simulink model "BatteryStoragePVPlantGFM"  (R2023a)
settings: Solver=FixedStepDiscrete  StartTime=0.0  StopTime=SimulationTime  RelTol=1e-3
PreLoadFcn:
  | run('BatteryStoragePVPlantGFMParameters')
undefined symbols (not defined in the file): Array, Base, battery, BatteryInverter, DiscIntNeverNeededParam, ee, Feeder, fRT, GFLBatteryController, GFMBatteryController, Grid, GridTransformer, Line, Load, Load2CB_final, Load2CB_initial, LVRT, maxSoC, maxVdc, minIrrad, minSoC, minVdc, Mpp, olTime, Panel, PVController, PVInverter, PVTransformer, Scenario, SM, SubTransmissionLine, Ts, VSMbase
libraries: ee_lib x51, nesl_utility x45, fl_lib x26, eeGeneralControl x18, simulink x12, eeTransforms x11, slpidlib x8, eePowerMeasurement x5, batteryecm_lib x2, eeTotalHarmonicDistorsion x2, spsLeadLagFilterLib x1, eeSmAC1C x1
(part 5 of 5)

== system BatteryStoragePVPlantGFM/BESS & PV PARK/60 MWhr Battery Energy Storage/Variant Subsystem/Grid Forming VSM/Battery Inverter B1/controller/GridFormingController/Current Limiting ==
  In Bus Element : Inport  PortName=measure  Element=Igd
  In Bus Element1 : Inport  PortName=measure  Element=Igq
  In Bus Element2 : Inport  Port=2  PortName=reactiveControl  Element=Vmd
  In Bus Element4 : Inport  Port=2  PortName=reactiveControl  Element=Vmq
  CurrentLimitingMethod : Subsystem  Variant=on  VariantControlMode=label  VariantControl=Choice  LabelModeActiveChoice=virimp
  Gain1 : Gain  Gain=1/(power/(sqrt(3)*girdLineVoltage)*sqrt(2/3))
  Gain5 : Gain  Gain=1/(power/(sqrt(3)*girdLineVoltage)*sqrt(2/3))
  Subtract : Sum  Inputs=+-
  Subtract1 : Sum  Inputs=-+
  Out Bus Element : Outport  PortName=currentLimiting  Element=Vmd
  Out Bus Element1 : Outport  PortName=currentLimiting  Element=Vmq
  Out Bus Element2 : Outport  PortName=currentLimiting  Element=Idmax
  Out Bus Element3 : Outport  PortName=currentLimiting  Element=Iqmax
  wires:
  In Bus Element/1 -> Gain5/1
  In Bus Element2/1 -> Subtract/1
  Gain1/1 -> CurrentLimitingMethod/2(Igq)
  In Bus Element4/1 -> Subtract1/2
  Subtract/1 -> Out Bus Element/1
  Subtract1/1 -> Out Bus Element1/1
  CurrentLimitingMethod/3(Idmax) -> Out Bus Element2/1
  CurrentLimitingMethod/4(Iqmax) -> Out Bus Element3/1
  Gain5/1 -> CurrentLimitingMethod/1(Igd)  "Q"
  In Bus Element1/1 -> Gain1/1
  CurrentLimitingMethod/1(delVmd) -> Subtract/2
  CurrentLimitingMethod/2(delVmq) -> Subtract1/1

== system BatteryStoragePVPlantGFM/BESS & PV PARK/60 MWhr Battery Energy Storage/Variant Subsystem/Grid Forming VSM/Battery Inverter B1/controller/GridFormingController/Measurement ==
  Vgabcc : Inport
  Igabc : Inport  Port=2
  Angle : Inport  Port=3
  Gain1 : Gain  Gain=1/power
  Gain2 : Gain  Gain=1/power
  Power Measurement (Three-Phase) : eePowerMeasurement/Power Measurement (Three-Phase)  LabelModeActiveChoice=Discrete  F=powerFreq  K=[1]  Seq=Positive  Ts=Ts
  abc2dq : Subsystem
  Out Bus Element : Outport  PortName=measure  Element=P
  Out Bus Element1 : Outport  PortName=measure  Element=Q
  Out Bus Element2 : Outport  PortName=measure  Element=Vgd
  Out Bus Element3 : Outport  PortName=measure  Element=Vgq
  Out Bus Element4 : Outport  PortName=measure  Element=Igd
  Out Bus Element5 : Outport  PortName=measure  Element=Igq
  Pmeas : Outport  Port=2
  Qmeas : Outport  Port=3
  wires:
  Vgabcc/1 -> abc2dq/3(Vgabc), Power Measurement (Three-Phase)/1
  Angle/1 -> abc2dq/2(Angle)
  Power Measurement (Three-Phase)/1 -> Gain2/1
  Igabc/1 -> abc2dq/1(Igabc), Power Measurement (Three-Phase)/2
  Power Measurement (Three-Phase)/2 -> Gain1/1
  Gain2/1 -> Pmeas/1, Out Bus Element/1  "Q"
  Gain1/1 -> Qmeas/1, Out Bus Element1/1  "Q"
  abc2dq/1(Vgd) -> Out Bus Element2/1  "Vgd"
  abc2dq/2(Vgq) -> Out Bus Element3/1  "Vgq"
  abc2dq/3(Igd) -> Out Bus Element4/1  "Igd"
  abc2dq/4(Igq) -> Out Bus Element5/1  "Igq"

== system BatteryStoragePVPlantGFM/BESS & PV PARK/60 MWhr Battery Energy Storage/Variant Subsystem/Grid Forming VSM/Battery Inverter B1/controller/GridFormingController/Power Control ==
  note: Reactive Power Control
  note: Active Power Control
  Pref : Inport
  In Bus Element2 : Inport  Port=2  PortName=measure  Element=P
  In Bus Element3 : Inport  Port=2  PortName=measure  Element=Q
  Qref : Inport  Port=3
  ActivePowerControl : Subsystem  Variant=on  VariantControlMode=label  VariantControl=Choice  LabelModeActiveChoice=vsm
  ReactiveControl : Subsystem
  Out Bus Element : Outport  PortName=reactiveControl  Element=Vmd
  Out Bus Element1 : Outport  PortName=reactiveControl  Element=Vmq
  Out Bus Element6 : Outport  Port=2  PortName=activeControl  Element=angle
  Out Bus Element4 : Outport  Port=2  PortName=activeControl  Element=w
  angle : Outport  Port=3
  wires:
  ActivePowerControl/2(w) -> Out Bus Element4/1
  In Bus Element2/1 -> ActivePowerControl/2(Pe)
  In Bus Element3/1 -> ReactiveControl/2(Qe)
  ActivePowerControl/1(Theta) -> angle/1, Out Bus Element6/1
  ReactiveControl/1(Vd) -> Out Bus Element/1
  ReactiveControl/2(Vq) -> Out Bus Element1/1
  Pref/1 -> ActivePowerControl/1(Pref)  "Q"
  Qref/1 -> ReactiveControl/1(Qref)  "Q"

== system BatteryStoragePVPlantGFM/BESS & PV PARK/60 MWhr Battery Energy Storage/Variant Subsystem/Grid Forming VSM/Battery Inverter B1/controller/GridFormingController/VoltageCurrentControl ==
  In Bus Element : Inport  PortName=currentLimiting  Element=Vmd
  In Bus Element1 : Inport  PortName=currentLimiting  Element=Vmq
  In Bus Element6 : Inport  PortName=currentLimiting  Element=Idmax
  In Bus Element7 : Inport  PortName=currentLimiting  Element=Iqmax
  Bus Element In6 : Inport  Port=2  PortName=activeControl  Element=w
  Bus Element In1 : Inport  Port=2  PortName=activeControl  Element=angle
  In Bus Element2 : Inport  Port=3  PortName=measure  Element=Vgd
  In Bus Element3 : Inport  Port=3  PortName=measure  Element=Vgq
  In Bus Element4 : Inport  Port=3  PortName=measure  Element=Igd
  In Bus Element5 : Inport  Port=3  PortName=measure  Element=Igq
  Controller : Subsystem
  Modulation Signal : Subsystem
  mabc : Outport
  wires:
  Controller/2(Vq) -> Modulation Signal/2(Vq)
  Modulation Signal/1(mabc) -> mabc/1
  Controller/1(Vd) -> Modulation Signal/1(Vd)
  In Bus Element4/1 -> Controller/6(Id)
  In Bus Element5/1 -> Controller/7(Iq)
  In Bus Element6/1 -> Controller/8(Idmax)
  In Bus Element7/1 -> Controller/9(Iqmax)
  In Bus Element2/1 -> Controller/4(Vsd)
  In Bus Element3/1 -> Controller/5(Vsq)
  Bus Element In6/1 -> Controller/1(Angfreq)
  In Bus Element/1 -> Controller/2(Vgdref)
  In Bus Element1/1 -> Controller/3(Vgqref)
  Bus Element In1/1 -> Modulation Signal/3(Angle)

== system BatteryStoragePVPlantGFM/BESS & PV PARK/60 MWhr Battery Energy Storage/Variant Subsystem/Grid Forming VSM/Battery Inverter B1/controller/GridFormingController/Current Limiting/CurrentLimitingMethod ==
  Igd : Inport
  Igq : Inport  Port=2
  currentLimitAndVirtual : Subsystem  VariantControl=both
  currentSaturation : Subsystem  VariantControl=ctSat
  virtualImpedance : Subsystem  VariantControl=virimp
  delVmd : Outport
  delVmq : Outport  Port=2
  Idmax : Outport  Port=3
  Iqmax : Outport  Port=4

== system BatteryStoragePVPlantGFM/BESS & PV PARK/60 MWhr Battery Energy Storage/Variant Subsystem/Grid Forming VSM/Battery Inverter B1/controller/GridFormingController/Measurement/abc2dq ==
  Igabc : Inport
  Angle : Inport  Port=2
  Vgabc : Inport  Port=3
  Supply Current to dq : Subsystem
  Supply Voltage  to dq1 : Subsystem
  Vgd : Outport
  Vgq : Outport  Port=2
  Igd : Outport  Port=3
  Igq : Outport  Port=4
  wires:
  Angle/1 -> Supply Voltage  to dq1/1(Angle), Supply Current to dq/2(Angle)
  Vgabc/1 -> Supply Voltage  to dq1/2(abc)
  Igabc/1 -> Supply Current to dq/1(abc)
  Supply Current to dq/1(Igd) -> Igd/1  "Id"
  Supply Current to dq/2(Igq) -> Igq/1  "Iq"
  Supply Voltage  to dq1/1(Vgd) -> Vgd/1  "Vgd"
  Supply Voltage  to dq1/2(Vgq) -> Vgq/1  "Vgq"

== system BatteryStoragePVPlantGFM/BESS & PV PARK/60 MWhr Battery Energy Storage/Variant Subsystem/Grid Forming VSM/Battery Inverter B1/controller/GridFormingController/Power Control/ActivePowerControl ==
  Pref : Inport
  Pe : Inport  Port=2
  droopControl : Subsystem  VariantControl=droop
  vsmControl : Subsystem  VariantControl=vsm
  Theta : Outport
  w : Outport  Port=2

== system BatteryStoragePVPlantGFM/BESS & PV PARK/60 MWhr Battery Energy Storage/Variant Subsystem/Grid Forming VSM/Battery Inverter B1/controller/GridFormingController/Power Control/ReactiveControl ==
  Qref : Inport
  Qe : Inport  Port=2
  Constant1 : Constant  Value=0
  Gain1 : Gain  Gain=girdLineVoltage*sqrt(2/3)
  Gain3 : Gain  Gain=girdLineVoltage*sqrt(2/3)
  Kq : Gain  Gain=QVoltDroop
  Low-Pass Filter (Discrete or Continuous) : eeGeneralControl/Low-Pass Filter (Discrete or Continuous)  K=1  T=QVoltFilterTC  B=inf  A=-inf  init_option=Specify as parameter  x0=0  Ts=activePowerSampleTime
  Saturation : Saturate  UpperLimit=1  LowerLimit=-1
  Sum : Sum  Inputs=|+-
  Sum1 : Sum  Inputs=|++
  V_ref : Constant  Value=GFMBatteryController.V_ref  SampleTime=Ts
  Vd : Outport
  Vq : Outport  Port=2
  wires:
  V_ref/1 -> Sum1/2
  Sum/1 -> Kq/1
  Kq/1 -> Saturation/1
  Qe/1 -> Low-Pass Filter (Discrete or Continuous)/1
  Constant1/1 -> [Vgqref]
  Low-Pass Filter (Discrete or Continuous)/1 -> Sum/2
  Saturation/1 -> Sum1/1
  Gain3/1 -> Vd/1  "Q"
  Gain1/1 -> Vq/1  "Q"
  Sum1/1 -> Gain3/1
  [Vgqref] -> Gain1/1
  Qref/1 -> Sum/1

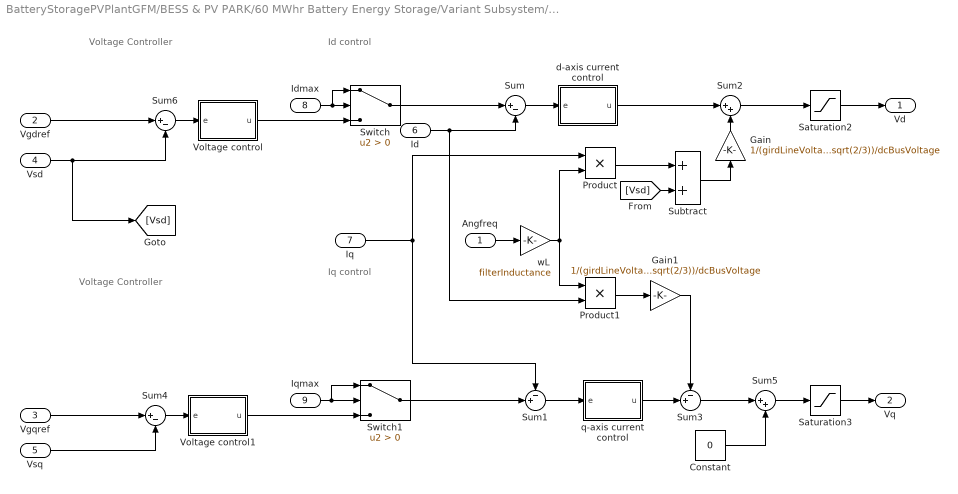
== system BatteryStoragePVPlantGFM/BESS & PV PARK/60 MWhr Battery Energy Storage/Variant Subsystem/Grid Forming VSM/Battery Inverter B1/controller/GridFormingController/VoltageCurrentControl/Controller ==
  note: Id control
  note: Voltage Controller
  note: Iq control
  note: Voltage Controller
  Angfreq : Inport
  Vgdref : Inport  Port=2
  Vgqref : Inport  Port=3
  Vsd : Inport  Port=4
  Vsq : Inport  Port=5
  Id : Inport  Port=6
  Iq : Inport  Port=7
  Idmax : Inport  Port=8
  Iqmax : Inport  Port=9
  Constant : Constant  Value=0
  Gain : Gain  Gain=1/(girdLineVoltage*sqrt(2/3))/dcBusVoltage
  Gain1 : Gain  Gain=1/(girdLineVoltage*sqrt(2/3))/dcBusVoltage
  Product : Product
  Product1 : Product
  Saturation2 : Saturate  UpperLimit=4  LowerLimit=-3
  Saturation3 : Saturate  UpperLimit=3  LowerLimit=-3
  Subtract : Sum
  Sum : Sum  Inputs=|+-
  Sum1 : Sum  Inputs=-+|
  Sum2 : Sum  Inputs=|++
  Sum3 : Sum  Inputs=-+|
  Sum4 : Sum  Inputs=|+-
  Sum5 : Sum  Inputs=|++
  Sum6 : Sum  Inputs=|+-
  Switch : Switch  Criteria=u2 > Threshold  SaturateOnIntegerOverflow=off  InputSameDT=off
  Switch1 : Switch  Criteria=u2 > Threshold  SaturateOnIntegerOverflow=off  InputSameDT=off
  Voltage control : Subsystem
  Voltage control1 : Subsystem
  d-axis current control : Subsystem
  q-axis current control : Subsystem
  wL : Gain  Gain=filterInductance
  Vd : Outport  VectorParamsAs1DForOutWhenUnconnected=off
  Vq : Outport  Port=2  VectorParamsAs1DForOutWhenUnconnected=off
  wires:
  Sum1/1 -> q-axis current control/1(e)
  wL/1 -> Product/2, Product1/1
  Iq/1 -> Sum1/1, Product/1
  Angfreq/1 -> wL/1
  Constant/1 -> Sum5/2
  Sum/1 -> d-axis current control/1(e)
  Saturation3/1 -> Vq/1
  Saturation2/1 -> Vd/1
  Product1/1 -> Gain1/1
  Product/1 -> Subtract/1
  [Vsd] -> Subtract/2
  Subtract/1 -> Gain/1
  Sum4/1 -> Voltage control1/1(e)
  Vgqref/1 -> Sum4/1
  Vsd/1 -> Sum6/2, [Vsd]
  d-axis current control/1(u) -> Sum2/1
  Sum2/1 -> Saturation2/1
  q-axis current control/1(u) -> Sum3/2
  Sum3/1 -> Sum5/1
  Sum5/1 -> Saturation3/1
  Gain1/1 -> Sum3/1
  Gain/1 -> Sum2/2
  Vgdref/1 -> Sum6/1
  Vsq/1 -> Sum4/2
  Id/1 -> Product1/2, Sum/2
  Sum6/1 -> Voltage control/1(e)
  Switch/1 -> Sum/1
  Idmax/1 -> Switch/1, Switch/2
  Switch1/1 -> Sum1/2
  Iqmax/1 -> Switch1/1, Switch1/2
  Voltage control/1(u) -> Switch/3
  Voltage control1/1(u) -> Switch1/3

== system BatteryStoragePVPlantGFM/BESS & PV PARK/60 MWhr Battery Energy Storage/Variant Subsystem/Grid Forming VSM/Battery Inverter B1/controller/GridFormingController/VoltageCurrentControl/Modulation Signal ==
  Vd : Inport
  Vq : Inport  Port=2
  Angle : Inport  Port=3
  Constant : Constant  Value=0
  Inverse Park Transform : eeTransforms/Inverse Park Transform  AxisAlignment=D-axis  PowerInvariant=off
  Mux1 : Mux  Inputs=3
  Saturation2 : Saturate  UpperLimit=1  LowerLimit=-1
  mabc : Outport  VectorParamsAs1DForOutWhenUnconnected=off
  wires:
  Inverse Park Transform/1 -> Saturation2/1
  Mux1/1 -> Inverse Park Transform/1
  Angle/1 -> Inverse Park Transform/2
  Saturation2/1 -> mabc/1
  Constant/1 -> Mux1/3
  Vd/1 -> Mux1/1
  Vq/1 -> Mux1/2

== system BatteryStoragePVPlantGFM/BESS & PV PARK/60 MWhr Battery Energy Storage/Variant Subsystem/Grid Forming VSM/Battery Inverter B1/controller/GridFormingController/Current Limiting/CurrentLimitingMethod/currentLimitAndVirtual ==
  Igd : Inport
  Igq : Inport  Port=2
  Constant2 : Constant  Value=0
  Constant3 : Constant  Value=0
  CurrentLimiting : Stateflow chart  TreatAsAtomicUnit=on
  delVmd : Outport
  delVmq : Outport  Port=2
  Idmax : Outport  Port=3
  Iqmax : Outport  Port=4
  wires:
  Igd/1 -> ?
  Igq/1 -> ?
  Constant2/1 -> Idmax/1
  Constant3/1 -> Iqmax/1

== system BatteryStoragePVPlantGFM/BESS & PV PARK/60 MWhr Battery Energy Storage/Variant Subsystem/Grid Forming VSM/Battery Inverter B1/controller/GridFormingController/Current Limiting/CurrentLimitingMethod/currentSaturation ==
  note: Vs-delV
  Igd : Inport
  Igq : Inport  Port=2
  Compare : Subsystem
  Constant : Constant  Value=maxCurrentLimit
  Constant1 : Constant  Value=0
  Constant2 : Constant  Value=0
  If : If
  If Action Subsystem : Subsystem  TreatAsAtomicUnit=on
  If Action Subsystem1 : Subsystem  TreatAsAtomicUnit=on
  Math Function : Math  Operator=hypot
  Merge : Merge
  Merge1 : Merge
  Subtract : Sum  Inputs=+-
  delVmd : Outport
  delVmq : Outport  Port=2
  Idmax : Outport  Port=3
  Iqmax : Outport  Port=4
  wires:
  Igd/1 -> [Isd], Math Function/1
  Igq/1 -> [Isq], Math Function/2
  Constant/1 -> Subtract/1
  Math Function/1 -> [Is], Subtract/2
  If/1 -> If Action Subsystem/Action
  [Isd] -> If Action Subsystem/2(Isd)
  [Isq] -> If Action Subsystem/3(Isq)
  Subtract/1 -> Compare/1(u)
  Compare/1(Out1) -> If/1
  If/2 -> If Action Subsystem1/Action
  [Is] -> If Action Subsystem/1(Is)
  If Action Subsystem/1(Idmax) -> Merge/1
  If Action Subsystem1/1(Idmax) -> Merge/2
  If Action Subsystem/2(Iqmax) -> Merge1/1
  If Action Subsystem1/2(Iqmax) -> Merge1/2
  Constant2/1 -> delVmq/1
  Constant1/1 -> delVmd/1
  Merge/1 -> Idmax/1
  Merge1/1 -> Iqmax/1

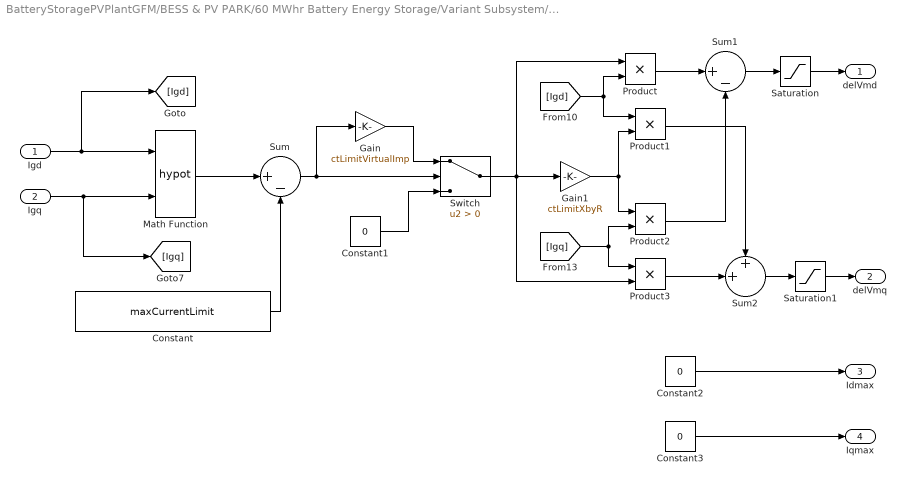
== system BatteryStoragePVPlantGFM/BESS & PV PARK/60 MWhr Battery Energy Storage/Variant Subsystem/Grid Forming VSM/Battery Inverter B1/controller/GridFormingController/Current Limiting/CurrentLimitingMethod/virtualImpedance ==
  Igd : Inport
  Igq : Inport  Port=2
  Constant : Constant  Value=maxCurrentLimit
  Constant1 : Constant  Value=0
  Constant2 : Constant  Value=0
  Constant3 : Constant  Value=0
  Gain : Gain  Gain=ctLimitVirtualImp
  Gain1 : Gain  Gain=ctLimitXbyR
  Math Function : Math  Operator=hypot
  Product{,1..3} (4 alike) : Product
  Saturation : Saturate  UpperLimit=1  LowerLimit=-1
  Saturation1 : Saturate  UpperLimit=1  LowerLimit=-1
  Sum : Sum  Inputs=|+-
  Sum1 : Sum  Inputs=|+-
  Sum2 : Sum  Inputs=++|
  Switch : Switch  Criteria=u2 > Threshold  SaturateOnIntegerOverflow=off  InputSameDT=off
  delVmd : Outport
  delVmq : Outport  Port=2
  Idmax : Outport  Port=3
  Iqmax : Outport  Port=4
  wires:
  Saturation/1 -> delVmd/1
  Sum/1 -> Gain/1, Switch/2
  Sum2/1 -> Saturation1/1
  Product3/1 -> Sum2/2
  Igq/1 -> [Igq], Math Function/2
  Product1/1 -> Sum2/1
  Gain1/1 -> Product1/2, Product2/1
  Sum1/1 -> Saturation/1
  Product/1 -> Sum1/1
  Product2/1 -> Sum1/2
  Constant/1 -> Sum/2
  Math Function/1 -> Sum/1
  [Igq] -> Product3/1, Product2/2
  Switch/1 -> Product3/2, Product/1, Gain1/1
  [Igd] -> Product1/1, Product/2
  Constant2/1 -> Idmax/1
  Constant3/1 -> Iqmax/1
  Gain/1 -> Switch/1
  Constant1/1 -> Switch/3
  Igd/1 -> Math Function/1, [Igd]
  Saturation1/1 -> delVmq/1

== system BatteryStoragePVPlantGFM/BESS & PV PARK/60 MWhr Battery Energy Storage/Variant Subsystem/Grid Forming VSM/Battery Inverter B1/controller/GridFormingController/Measurement/abc2dq/Supply Current to dq ==
  abc : Inport
  Angle : Inport  Port=2
  Demux : Demux  Outputs=3
  Park Transform : eeTransforms/Park Transform  AxisAlignment=D-axis  PowerInvariant=off
  Terminator : Terminator
  Igd : Outport  VectorParamsAs1DForOutWhenUnconnected=off
  Igq : Outport  Port=2  VectorParamsAs1DForOutWhenUnconnected=off
  wires:
  Demux/3 -> Terminator/1
  Park Transform/1 -> Demux/1
  Demux/2 -> Igq/1
  Demux/1 -> Igd/1
  abc/1 -> Park Transform/1
  Angle/1 -> Park Transform/2

== system BatteryStoragePVPlantGFM/BESS & PV PARK/60 MWhr Battery Energy Storage/Variant Subsystem/Grid Forming VSM/Battery Inverter B1/controller/GridFormingController/Measurement/abc2dq/Supply Voltage  to dq1 ==
  Angle : Inport
  abc : Inport  Port=2
  Demux : Demux  Outputs=3
  Park Transform : eeTransforms/Park Transform  AxisAlignment=D-axis  PowerInvariant=off
  Terminator : Terminator
  Vgd : Outport  VectorParamsAs1DForOutWhenUnconnected=off
  Vgq : Outport  Port=2  VectorParamsAs1DForOutWhenUnconnected=off
  wires:
  Demux/3 -> Terminator/1
  Park Transform/1 -> Demux/1
  Demux/2 -> Vgq/1
  Demux/1 -> Vgd/1
  abc/1 -> Park Transform/1
  Angle/1 -> Park Transform/2

== system BatteryStoragePVPlantGFM/BESS & PV PARK/60 MWhr Battery Energy Storage/Variant Subsystem/Grid Forming VSM/Battery Inverter B1/controller/GridFormingController/Power Control/ActivePowerControl/droopControl ==
  Pref : Inport
  Pe : Inport  Port=2
  Add : Sum  Inputs=+-
  Constant : Constant
  Constant5 : Constant  Value=pi/2
  Gain : Gain  Gain=powerFreq*2*pi
  Integrator1 : Integrator  WrapState=on  WrappedStateUpperValue=2*pi  WrappedStateLowerValue=0
  Lead-Lag Filter : spsLeadLagFilterLib/Lead-Lag Filter  T1=droopT1  T2=droopT2  Vdc_Init=0  Ts=activePowerSampleTime
  Low-Pass Filter (Discrete or Continuous) : eeGeneralControl/Low-Pass Filter (Discrete or Continuous)  K=1  T=droopTC  B=inf  A=-inf  init_option=Specify as parameter  x0=0  Ts=activePowerSampleTime
  Scope : Scope
  Scope1 : Scope
  Scope2 : Scope  NumInputPorts=2
  Scope3 : Scope  NumInputPorts=2
  Sum : Sum  Inputs=|-+
  Sum1 : Sum  Inputs=|-+
  mp : Gain  Gain=droopSlope
  Theta : Outport
  w : Outport  Port=2
  wires:
  Low-Pass Filter (Discrete or Continuous)/1 -> Sum1/1
  mp/1 -> Low-Pass Filter (Discrete or Continuous)/1
  Sum/1 -> Scope/1, mp/1
  Constant/1 -> Sum1/2
  Pe/1 -> Scope2/2, Lead-Lag Filter/1
  Integrator1/1 -> Add/1
  Lead-Lag Filter/1 -> Scope2/1, Sum/2
  Sum1/1 -> Gain/1
  Add/1 -> Theta/1
  Constant5/1 -> Add/2
  Pref/1 -> Scope1/1, Sum/1
  Gain/1 -> Scope3/1, w/1, Scope3/2, Integrator1/1

== system BatteryStoragePVPlantGFM/BESS & PV PARK/60 MWhr Battery Energy Storage/Variant Subsystem/Grid Forming VSM/Battery Inverter B1/controller/GridFormingController/Power Control/ActivePowerControl/vsmControl ==
  Pref : Inport
  Pe : Inport  Port=2
  1/2H : Gain  Gain=1/vsmInertiaTC
  Add : Sum  Inputs=+-
  Constant2 : Constant  Value=pi/2
  Discrete-Time Integrator : DiscreteIntegrator  IntegratorMethod=Integration: Backward Euler  InitialCondition=1  SampleTime=activePowerSampleTime  LimitOutput=on  UpperSaturationLimit=1.1  LowerSaturationLimit=0.9  ICPrevOutput=DiscIntNeverNeededParam  ICPrevScaledInput=DiscIntNeverNeededParam
  Gain : Gain  Gain=powerFreq*2*pi
  Gain2 : Gain  Gain=vsmDampingConst*powerFreq*2*pi
  Integrator with Wrapped State (Discrete or Continuous) : eeGeneralControl/Integrator with Wrapped State (Discrete or Continuous)  LabelModeActiveChoice=Discrete  WrappedStateUpperValue=2*pi  WrappedStateLowerValue=0  x0=0  Ts=Ts
      settings: LibrarySourceBlock=|
      | ee_sl_lib/General Control/Integrator with
      | Wrapped State
      | (Discrete or Continuous)
  Kp : Gain  Gain=vsmFreqDroop
  Low-Pass Filter (Discrete or Continuous) : eeGeneralControl/Low-Pass Filter (Discrete or Continuous)  K=1  T=vsmPmeasFilterTC  B=inf  A=-inf  init_option=Specify as parameter  x0=0  Ts=activePowerSampleTime
  Sum : Sum  Inputs=|+-
  Sum1 : Sum  Inputs=-+-|
  Sum2 : Sum  Inputs=|+-
  Sum3 : Sum  Inputs=++|
  Unit Delay : UnitDelay  InitialCondition=0.98  SampleTime=1e-6  HasFrameUpgradeWarning=on
  Unit Delay1 : UnitDelay  InitialCondition=0.98  SampleTime=1e-6  HasFrameUpgradeWarning=on
  w_ref : Constant  Value=GFMBatteryController.w_ref  SampleTime=Ts
  Theta : Outport
  w : Outport  Port=2
  wires:
  Integrator with Wrapped State (Discrete or Continuous)/1 -> Add/1
  Sum1/1 -> 1/2H/1
  Sum/1 -> Kp/1
  Constant2/1 -> Add/2
  Add/1 -> Theta/1
  w_ref/1 -> Sum2/2, Sum/1
  Pe/1 -> Low-Pass Filter (Discrete or Continuous)/1
  Low-Pass Filter (Discrete or Continuous)/1 -> Sum1/1
  Kp/1 -> Sum3/2
  Pref/1 -> Sum3/1
  Gain2/1 -> Sum1/3
  Sum3/1 -> Sum1/2
  Sum2/1 -> Gain2/1
  1/2H/1 -> Discrete-Time Integrator/1
  Gain/1 -> Integrator with Wrapped State (Discrete or Continuous)/1, w/1
  Discrete-Time Integrator/1 -> Gain/1, Unit Delay/1, Unit Delay1/1
  Unit Delay/1 -> Sum2/1
  Unit Delay1/1 -> Sum/2

== system BatteryStoragePVPlantGFM/BESS & PV PARK/60 MWhr Battery Energy Storage/Variant Subsystem/Grid Forming VSM/Battery Inverter B1/controller/GridFormingController/VoltageCurrentControl/Controller/Voltage control ==
  e : Inport
  Discrete-Time Integrator : DiscreteIntegrator  IntegratorMethod=Integration: Backward Euler  SampleTime=voltControlTs  LimitOutput=on  UpperSaturationLimit=(power/(sqrt(3)*girdLineVoltage))*sqrt(2/3)*1.5  LowerSaturationLimit=(power/(sqrt(3)*girdLineVoltage))*sqrt(2/3)*-1.5  ICPrevOutput=DiscIntNeverNeededParam  ICPrevScaledInput=DiscIntNeverNeededParam
  Ki : Gain  Gain=VdIGain
  Kp : Gain  Gain=vdPGain
  Saturation : Saturate  UpperLimit=(power/(sqrt(3)*girdLineVoltage))*sqrt(2/3)*1.5  LowerLimit=(power/(sqrt(3)*girdLineVoltage))*sqrt(2/3)*-1.5
  Sum7 : Sum  Inputs=|++
  u : Outport  VectorParamsAs1DForOutWhenUnconnected=off
  wires:
  Discrete-Time Integrator/1 -> Sum7/2
  Sum7/1 -> Saturation/1
  e/1 -> Ki/1, Kp/1
  Kp/1 -> Sum7/1
  Saturation/1 -> u/1
  Ki/1 -> Discrete-Time Integrator/1

== system BatteryStoragePVPlantGFM/BESS & PV PARK/60 MWhr Battery Energy Storage/Variant Subsystem/Grid Forming VSM/Battery Inverter B1/controller/GridFormingController/VoltageCurrentControl/Controller/Voltage control1 ==
  e : Inport
  Discrete-Time Integrator : DiscreteIntegrator  IntegratorMethod=Integration: Backward Euler  SampleTime=voltControlTs  LimitOutput=on  UpperSaturationLimit=(power/(sqrt(3)*girdLineVoltage))*sqrt(2/3)*1.5  LowerSaturationLimit=(power/(sqrt(3)*girdLineVoltage))*sqrt(2/3)*-1.5  ICPrevOutput=DiscIntNeverNeededParam  ICPrevScaledInput=DiscIntNeverNeededParam
  Ki : Gain  Gain=VqIGain
  Kp : Gain  Gain=VqPGain
  Saturation : Saturate  UpperLimit=(power/(sqrt(3)*girdLineVoltage))*sqrt(2/3)*1.5  LowerLimit=(power/(sqrt(3)*girdLineVoltage))*sqrt(2/3)*-1.5
  Sum7 : Sum  Inputs=|++
  u : Outport  VectorParamsAs1DForOutWhenUnconnected=off
  wires:
  Discrete-Time Integrator/1 -> Sum7/2
  Sum7/1 -> Saturation/1
  e/1 -> Ki/1, Kp/1
  Kp/1 -> Sum7/1
  Ki/1 -> Discrete-Time Integrator/1
  Saturation/1 -> u/1

== system BatteryStoragePVPlantGFM/BESS & PV PARK/60 MWhr Battery Energy Storage/Variant Subsystem/Grid Forming VSM/Battery Inverter B1/controller/GridFormingController/VoltageCurrentControl/Controller/d-axis current control ==
  e : Inport
  Discrete-Time Integrator : DiscreteIntegrator  IntegratorMethod=Integration: Backward Euler  SampleTime=currentControlTs  LimitOutput=on  UpperSaturationLimit=10  LowerSaturationLimit=-10  ICPrevOutput=DiscIntNeverNeededParam  ICPrevScaledInput=DiscIntNeverNeededParam
  Ki : Gain  Gain=IdIGain
  Kp : Gain  Gain=IdPGain
  Saturation : Saturate  UpperLimit=4  LowerLimit=-4
  Sum7 : Sum  Inputs=|++
  u : Outport  VectorParamsAs1DForOutWhenUnconnected=off
  wires:
  Discrete-Time Integrator/1 -> Sum7/2
  Sum7/1 -> Saturation/1
  e/1 -> Ki/1, Kp/1
  Kp/1 -> Sum7/1
  Saturation/1 -> u/1
  Ki/1 -> Discrete-Time Integrator/1

== system BatteryStoragePVPlantGFM/BESS & PV PARK/60 MWhr Battery Energy Storage/Variant Subsystem/Grid Forming VSM/Battery Inverter B1/controller/GridFormingController/VoltageCurrentControl/Controller/q-axis current control ==
  e : Inport
  Discrete-Time Integrator : DiscreteIntegrator  IntegratorMethod=Integration: Backward Euler  SampleTime=currentControlTs  LimitOutput=on  UpperSaturationLimit=10  LowerSaturationLimit=-10  ICPrevOutput=DiscIntNeverNeededParam  ICPrevScaledInput=DiscIntNeverNeededParam
  Ki : Gain  Gain=IqIGain
  Kp : Gain  Gain=IqPGain
  Saturation : Saturate  UpperLimit=3  LowerLimit=-3
  Sum7 : Sum  Inputs=|++
  u : Outport  VectorParamsAs1DForOutWhenUnconnected=off
  wires:
  Ki/1 -> Discrete-Time Integrator/1
  Kp/1 -> Sum7/1
  e/1 -> Ki/1, Kp/1
  Sum7/1 -> Saturation/1
  Saturation/1 -> u/1
  Discrete-Time Integrator/1 -> Sum7/2

== system BatteryStoragePVPlantGFM/BESS & PV PARK/60 MWhr Battery Energy Storage/Variant Subsystem/Grid Forming VSM/Battery Inverter B1/controller/GridFormingController/Current Limiting/CurrentLimitingMethod/currentSaturation/Compare ==
  u : Inport
  AND : Logic  IconShape=distinctive  AllPortsSameDT=off  OutDataTypeStr=boolean
  Compare To Constant : simulink/Logic and Bit Operations/Compare To Constant  relop=>  const=ctLimitDelayTime  OutDataTypeStr=boolean
  Compare To Zero : simulink/Logic and Bit Operations/Compare To Zero  relop=<=  OutDataTypeStr=boolean
  Data Type Conversion : DataTypeConversion  SaturateOnIntegerOverflow=off  RndMeth=Floor
  Data Type Conversion1 : DataTypeConversion  SaturateOnIntegerOverflow=off  RndMeth=Floor
  Integrator : Integrator
  Out1 : Outport
  wires:
  AND/1 -> Data Type Conversion/1
  Compare To Zero/1 -> Data Type Conversion1/1
  Compare To Constant/1 -> AND/2
  u/1 -> Compare To Zero/1
  Integrator/1 -> Compare To Constant/1
  Data Type Conversion/1 -> Out1/1
  Data Type Conversion1/1 -> Integrator/1, AND/1

== system BatteryStoragePVPlantGFM/BESS & PV PARK/60 MWhr Battery Energy Storage/Variant Subsystem/Grid Forming VSM/Battery Inverter B1/controller/GridFormingController/Current Limiting/CurrentLimitingMethod/currentSaturation/If Action Subsystem ==
  Is : Inport
  Isd : Inport  Port=2
  Isq : Inport  Port=3
  Action Port : ActionPort
  Constant : Constant  Value=ctLimitMaxCurrent
  Divide : Product  Inputs=*/
  Product : Product
  Product1 : Product
  Idmax : Outport
  Iqmax : Outport  Port=2
  wires:
  Product/1 -> ?
  Constant/1 -> Divide/1
  Is/1 -> Divide/2
  Divide/1 -> Product1/2, Product/1
  Isd/1 -> Product1/1
  Isq/1 -> Product/2
  Product1/1 -> Idmax/1

== system BatteryStoragePVPlantGFM/BESS & PV PARK/60 MWhr Battery Energy Storage/Variant Subsystem/Grid Forming VSM/Battery Inverter B1/controller/GridFormingController/Current Limiting/CurrentLimitingMethod/currentSaturation/If Action Subsystem1 ==
  Action Port : ActionPort
  Constant3 : Constant  Value=0
  Constant4 : Constant  Value=0
  Idmax : Outport
  Iqmax : Outport  Port=2
  wires:
  Constant4/1 -> Iqmax/1
  Constant3/1 -> Idmax/1

== stateflow chart BatteryStoragePVPlantGFM/BESS & PV PARK/60 MWhr Battery Energy Storage/Variant Subsystem/Grid Forming VSM/Battery Inverter B1/controller/GridFormingController/Current Limiting/CurrentLimitingMethod/currentLimitAndVirtual/CurrentLimiting ==
  state Mode2_BatCharge_pvMPPT
    entry:
    pvMPPT=1;
    BatCharge=1;
    modeNum=2;
    overload=0;
    exit:
    pvMPPT=0; BatCharge=0;
  state Start_Mode
    entry:
    ShutDown = 0;
    loadShutDown = 1;
    pvMPPT=0;
    VoltageControl=1;
    BatIsolate=1;
    modeNum=0;
    overload=0;
    exit:
    pvMPPT=0;
    BatIsolate=0;
    VoltageControl=0;
    loadShutDown = 0;
  state Mode5_System_ShutDown
    entry:
    PVoff=1; BatIsolate=1;
    ShutDown =1; modeNum=5;
    exit:
    ShutDown =0; PVoff=0;
    BatIsolate=0;
  state Mode1_batIsolated_pvVoltControl
    entry:
    VoltageControl=1; BatIsolate=1;
    modeNum=1;
    exit:
    VoltageControl=0; BatIsolate=0;
  state Mode6_pvMPPT_BatCharge_noload
    entry:
    pvMPPT=1; BatCharge=1;
    loadShutDown=1; modeNum=6;
    overload=1;
    exit:
    loadShutDown=0; pvMPPT=0;
    BatCharge=0;
  state Mode3_BatDischarge_pvMPPT
    entry:
    pvMPPT=1; BatDischarge=1;
    modeNum=3; overload=0;
    exit:
    pvMPPT=0;  BatDischarge=0;
  state Mode4_night_mode
    entry:
    PVoff=1; BatDischarge=1;
    modeNum=4;
    exit:
    PVoff=0; BatDischarge=0;
  Mode2_BatCharge_pvMPPT -> (junction 121) [order 3] : [Irrad<minIrrad && SoC>minSoC]
  Mode2_BatCharge_pvMPPT -> (junction 131) [order 2] : [Vdc < minVdc && SoC>minSoC]
  (junction 121) -> Mode4_night_mode
  (junction 131) -> (junction 154)
  Mode2_BatCharge_pvMPPT -> (junction 117) [order 5] : [Irrad<minIrrad && SoC<minSoC]
  (junction 132) -> Mode2_BatCharge_pvMPPT : [Vdc > maxVdc && Irrad>minIrrad]
  (junction 117) -> Mode5_System_ShutDown
  (junction 155) -> (junction 132)
  (junction 130) -> Mode2_BatCharge_pvMPPT : [(Irrad >minIrrad && overload==0) || ...
      | (overload==1 && rsflag==1)]
  Mode5_System_ShutDown -> (junction 130)
  Start_Mode -> Mode2_BatCharge_pvMPPT [order 1] : [SoC<minSoC]
  (junction 123) -> Mode2_BatCharge_pvMPPT
  Mode6_pvMPPT_BatCharge_noload -> (junction 123) [order 3] : [rsflag ==1 && Irrad > minIrrad  ...
      | && SoC <= minSoC]
  Mode2_BatCharge_pvMPPT -> (junction 125) [order 4]
  (default) -> Start_Mode
  (junction 125) -> Mode6_pvMPPT_BatCharge_noload : [duration(Vdc<minVdc)>olTime ...
      |  && SoC<minSoC]
  Mode2_BatCharge_pvMPPT -> Mode1_batIsolated_pvVoltControl [order 1] : [(SoC>maxSoC) || ...
      | (duration(Vdc>maxVdc)>olTime)]
  Start_Mode -> Mode3_BatDischarge_pvMPPT [order 2] : [SoC>minSoC]
  Mode1_batIsolated_pvVoltControl -> (junction 126)
  Mode6_pvMPPT_BatCharge_noload -> Mode5_System_ShutDown [order 2] : [(SoC<minSoC && ...
      | Irrad<minIrrad)|| ...
      | SoC>maxSoC]
  (junction 126) -> Mode3_BatDischarge_pvMPPT : [Vdc<minVdc]
  (junction 161) -> Mode5_System_ShutDown
  Mode4_night_mode -> Mode5_System_ShutDown [order 2] : [SoC<minSoC]
  Mode6_pvMPPT_BatCharge_noload -> (junction 127) [order 1] : [SoC>minSoC && rsflag==1]
  (junction 127) -> Mode3_BatDischarge_pvMPPT
  (junction 133) -> Mode6_pvMPPT_BatCharge_noload
  Mode3_BatDischarge_pvMPPT -> (junction 133) [order 2] : [(duration(Vdc<minVdc)>olTime || ...
      |  (SoC<minSoC && Vdc<minVdc)) && Irrad>minIrrad]
  Mode3_BatDischarge_pvMPPT -> (junction 161) [order 3] : [(SoC<minSoC && Irrad<minIrrad) || ( Irrad<minIrrad && duration(Vdc<minVdc)>olTime) ]
  Mode3_BatDischarge_pvMPPT -> (junction 155) [order 1]
  Mode4_night_mode -> Mode3_BatDischarge_pvMPPT [order 1] : [Irrad>minIrrad]
  Mode3_BatDischarge_pvMPPT -> Mode4_night_mode [order 4] : [Irrad<minIrrad && SoC>minSoC]
  (junction 154) -> Mode3_BatDischarge_pvMPPT
  data: Irrad input; Vdc input; SoC input; ShutDown output; maxSoC parameter; maxVdc parameter; minIrrad parameter; minSoC parameter; minVdc parameter; loadShutDown output; VoltageControl output; BatCharge output; BatDischarge output; BatIsolate output; PVoff output; pvMPPT output; modeNum output; rsflag input; overload output; olTime parameter
